simulink model "Combine4_Model"  (R2024b)
settings: Solver=VariableStepAuto  StartTime=0.0  StopTime=10.0  RelTol=1e-3
libraries: NSA_DEVS_SINKS x5, NSA_DEVS_SOURCES x4, NSA_DEVS_ROUTING x1, NSA_DEVS_LOGISTICS x1
settings Model: Creator=david  LastModifiedBy=peter
settings RTWCC: GPUComputeCapability=3.5

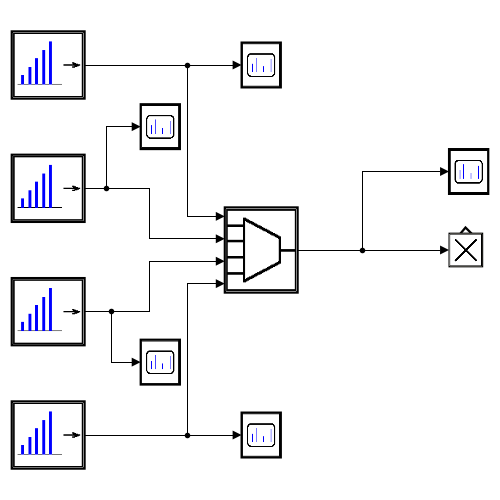
[thumbnail: Simulink's stored preview of the top-level diagram]
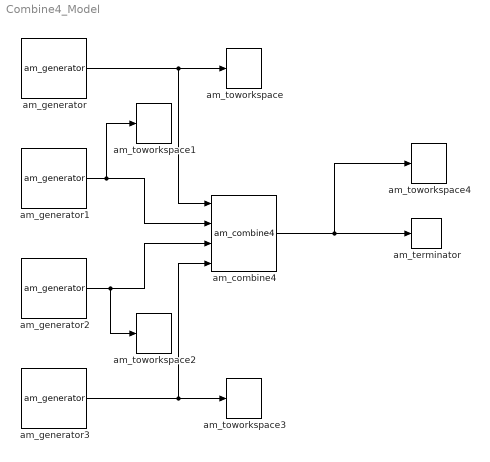
== system Combine4_Model ==
  am_combine4 : NSA_DEVS_ROUTING/am_combine4  tD=[0,10]  tau=[0,10]  debug=0
      settings: SourceProductName=Routing
  am_generator : NSA_DEVS_SOURCES/am_generator  tG=1  n0=1  nG=100  tD=[0,2]  debug=0
      settings: SourceProductName=Sources
  am_generator1 : NSA_DEVS_SOURCES/am_generator  tG=2  n0=21  nG=100  tD=[0,2]  debug=0
      settings: SourceProductName=Sources
  am_generator2 : NSA_DEVS_SOURCES/am_generator  tG=3  n0=41  nG=100  tD=[0,2]  debug=0
      settings: SourceProductName=Sources
  am_generator3 : NSA_DEVS_SOURCES/am_generator  tG=3.5  n0=12  nG=100  tD=[0,2]  debug=0
      settings: SourceProductName=Sources
  am_terminator : NSA_DEVS_LOGISTICS/am_terminator  tau=[0,1]  debug=0
      settings: SourceProductName=Logistics
  am_toworkspace : NSA_DEVS_SINKS/am_toworkspace  varname="\"gen1Out\""  t0=0  format="\"vector\""  tau=[0,1]  debug=0
      settings: SourceProductName=Sinks
  am_toworkspace1 : NSA_DEVS_SINKS/am_toworkspace  varname="\"gen2Out\""  t0=0  format="\"vector\""  tau=[0,1]  debug=0
      settings: SourceProductName=Sinks
  am_toworkspace2 : NSA_DEVS_SINKS/am_toworkspace  varname="\"gen3Out\""  t0=0  format="\"vector\""  tau=[0,1]  debug=0
      settings: SourceProductName=Sinks
  am_toworkspace3 : NSA_DEVS_SINKS/am_toworkspace  varname="\"gen4Out\""  t0=0  format="\"vector\""  tau=[0,1]  debug=0
      settings: SourceProductName=Sinks
  am_toworkspace4 : NSA_DEVS_SINKS/am_toworkspace  varname="\"combOut\""  t0=0  format="\"vector\""  tau=[0,1]  debug=0
      settings: SourceProductName=Sinks
  wires:
  am_generator1/1 -> am_toworkspace1/1, am_combine4/2
  am_generator2/1 -> am_toworkspace2/1, am_combine4/3
  am_generator/1 -> am_toworkspace/1, am_combine4/1
  am_generator3/1 -> am_toworkspace3/1, am_combine4/4
  am_combine4/1 -> am_toworkspace4/1, am_terminator/1
